simulink model "A1"  (R2019a)
settings: Solver=FixedStepAuto  StartTime=0.0  StopTime=20.0  RelTol=1e-3  EnableMultiTasking=on
libraries: arduinolib x1
settings Model: SimulationMode=external  ExtModeTrigDuration=2  Creator=timrehbronn  LastModifiedBy=timrehbronn
settings OptimizationCC: EnhancedBackFolding=on  PassReuseOutputArgsAs=Individual arguments  MaxStackSize=64  OptimizeBlockOrder=speed  DifferentSizesBufferReuse=on  OptimizationCustomize=off
settings DebuggingCC: ParameterTunabilityLossMsg=error
settings HardwareCC: ProdBitPerInt=16  ProdBitPerPointer=16  ProdBitPerSizeT=16  ProdBitPerPtrDiffT=16  ProdLargestAtomicFloat=None  ProdWordSize=8  ProdHWDeviceType=Atmel->AVR  UseEmbeddedCoderFeatures=off  UseSimulinkCoderFeatures=off
settings SFSimCC: MATLABDynamicMemAlloc=off
settings RTWCC: SystemTargetFile=ert.tlc  HardwareBoard=Arduino Mega 2560  TLCOptions=-aInlineSetEventsForThisBaseRateFcn=TLC_FALSE -aSuppressMultiTaskScheduler=TLC_FALSE -aRateBasedStepFcn=1  TemplateMakefile=ert_default_tmf  GenerateReport=on  Toolchain=Arduino AVR  BuildConfiguration=Faster Runs  IncludeHyperlinkInReport=on  LaunchReport=on  GenerateTraceInfo=on  GenerateTraceReport=on  GenerateTraceReportSl=on  GenerateTraceReportSf=on  GenerateTraceReportEml=on
settings CodeAppCC: ForceParamTrailComments=on  IgnoreCustomStorageClasses=off  OperatorAnnotations=on  SimulinkDataObjDesc=on  SFDataObjDesc=on  InsertBlockDesc=on
settings ERTTargetCC: SupportContinuousTime=on  SupportNonInlinedSFcns=on  SupportVariableSizeSignals=on  ExtModeStaticAllocSize=2048

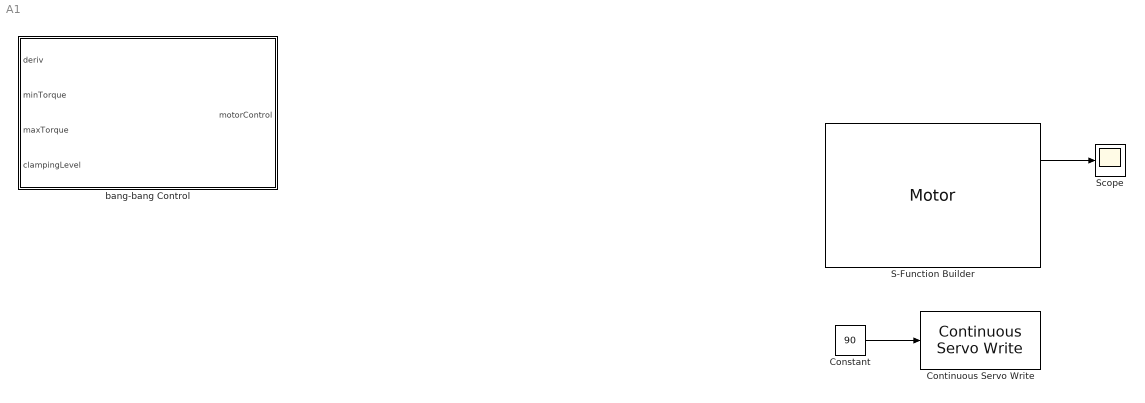
== system A1 ==
  Constant : Constant  Value=90
  Continuous Servo Write : arduinolib/Continuous Servo Write  pinNumber=2  ServoIndex=0  blockPlatform=ARDUINO
      settings: SourceProductName=Simulink Support Package for Arduino Hardware  SourceProductBaseCode=ARDUINO
  S-Function Builder : S-Function  InitFcn=try, set_param(gcb,'FunctionName','Motor'), end  FunctionName=Motor  SFunctionModules=Motor_wrapper  SFunctionDeploymentMode=off  EnableBusSupport=off  mask(S-Function Builder){}
      mask help: Simulink:masks:SFunctionBuilder_MD
      mask init:
      | val = [[.9  0.75 0.75 1 1 .9 .9 1]',[1 1 0.75 0.75 .9 .9 1 .9]'];try , sys = get_param(gcb,'SfunBuilderFcnName');if isempty(sys), sys = get_param(gcb,'FunctionName'); end,catch, sys = get_param(gcb,'FunctionName'); end
      settings: CopyFcn=set_param(gcbh,'LinkStatus','none')  PreSaveFcn=try, set_param(gcb,'FunctionName','Motor'), end  OpenFcn=sfunctionwizard(gcbh)
      mask Display: plot(val(:,1),val(:,2)),disp(sys), port_label('output',1,'posRad'), port_label('output',2,'deriv')
  Scope : Scope
  bang-bang Control : MATLAB Function  TreatAsAtomicUnit=on
  wires:
  S-Function Builder/1 -> Scope/1
  Constant/1 -> Continuous Servo Write/1

== matlab function A1/bang-bang Control ==
  data: deriv input; motorControl output; minTorque input; maxTorque input; clampingLevel input
function motorControl   = fcn(deriv,minTorque, maxTorque, clampingLevel)
    persistent  drive lastDeriv signDeriv clamping;
    if(isempty(drive))
        drive = int16(15);
        lastDeriv = 0;
        signDeriv = 0;
        clamping = 0;
    end

    if(deriv==0)
        if(~clamping)
            if(lastDeriv > 0)
                drive = int16(maxTorque);
            else
                drive = int16(minTorque);
            end
            clamping = 1;
            signDeriv = lastDeriv;
        end
    end
    
    if(clamping)
        if(signDeriv > 0 && deriv < (-1 * clampingLevel))
            clamping  = 0;
        elseif(signDeriv < 0 && deriv > clampingLevel)
            clamping = 0;
        end
    end
    
    lastDeriv = deriv;
    motorControl = double(drive);
